simulink model "RotationalPendulum_Linear_2021b2"  (R2021b)
settings: Solver=VariableStepAuto  StartTime=0.0  StopTime=10.0  RelTol=1e-3
libraries: cstblocks x1
settings Model: Creator=djangovanderplas  LastModifiedBy=thoma
settings DebuggingCC: UnconnectedInputMsg=none  UnconnectedOutputMsg=none  UnconnectedLineMsg=none
settings ModelReferenceCC: EnableRefExpFcnMdlSchedulingChecks=off
settings RTWCC: GPUComputeCapability=5.0  DLArmComputeVersion=20.02.1
settings ConfigComp: CovBoundaryAbsTol=1.0e-5

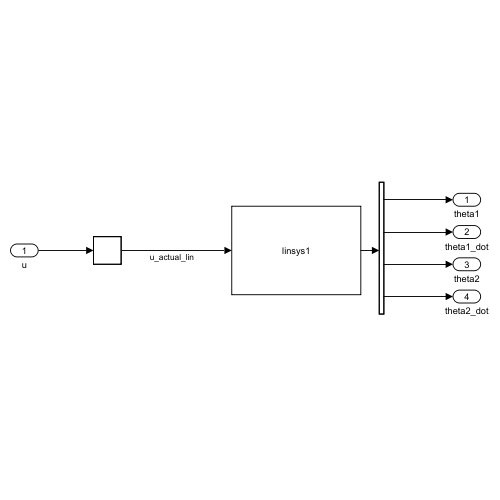
[thumbnail: Simulink's stored preview of the top-level diagram]
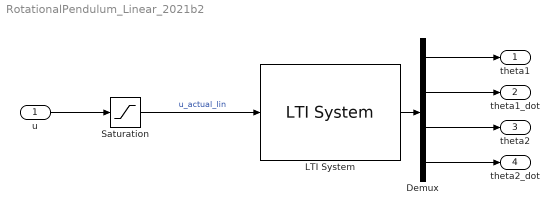
== system RotationalPendulum_Linear_2021b2 ==
  u : Inport
  Demux : Demux
  LTI System : cstblocks/LTI System  sys=linsys1  IC=x0
  Saturation : Saturate  UpperLimit=1  LowerLimit=-1
  theta1 : Outport
  theta1_dot : Outport  Port=2
  theta2 : Outport  Port=3
  theta2_dot : Outport  Port=4
  wires:
  u/1 -> Saturation/1
  LTI System/1 -> Demux/1
  Demux/1 -> theta1/1
  Demux/2 -> theta1_dot/1
  Demux/3 -> theta2/1
  Demux/4 -> theta2_dot/1
  Saturation/1 -> LTI System/1  "u_actual_lin"
